simulink model "threeDOF"  (R2026a)
settings: Solver=FixedStepAuto  StopTime=30  FixedStep=0.01
settings Model: Creator=Lenovo  LastModifiedBy=Lenovo

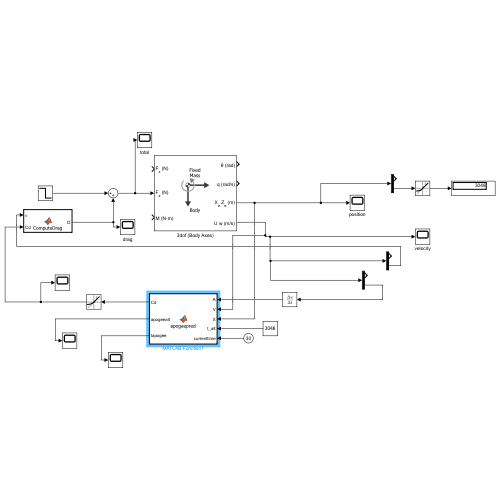
[thumbnail: Simulink's stored preview of the top-level diagram]
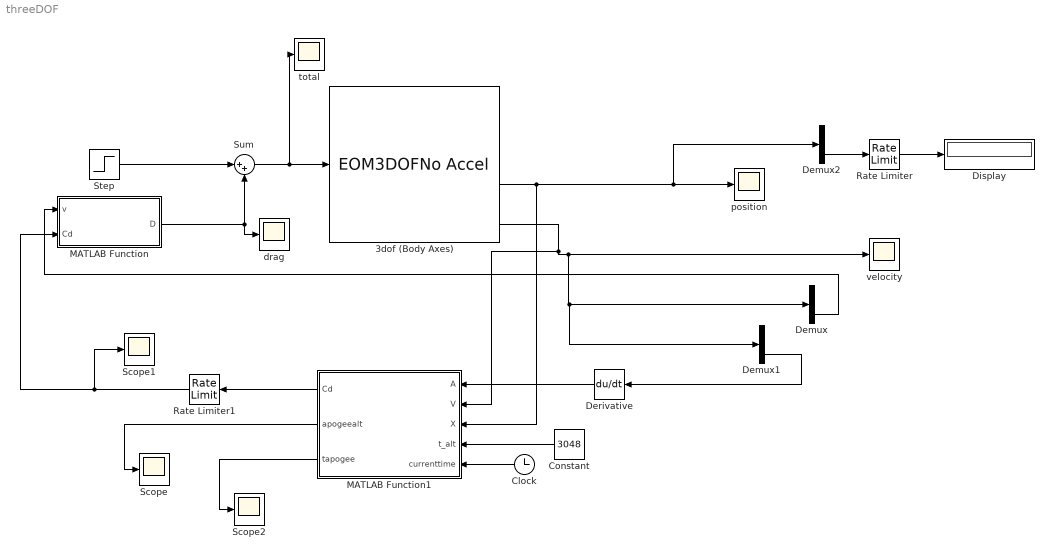
== system threeDOF ==
  3dof (Body Axes) : EOM3DOFNoAccel  v_ini=0  mass=19  g=-9.81
  Clock : Clock
  Constant : Constant  Value=3048
  Demux : Demux  Outputs=2
  Demux1 : Demux  Outputs=2
  Demux2 : Demux  Outputs=2
  Derivative : Derivative
  Display : Display
  MATLAB Function : MATLAB Function  TreatAsAtomicUnit=on
  MATLAB Function1 : MATLAB Function  TreatAsAtomicUnit=on
  Rate Limiter : RateLimiter  RisingSlewLimit=99999  FallingSlewLimit=0  SampleTimeMode=inherited
  Rate Limiter1 : RateLimiter  RisingSlewLimit=2  FallingSlewLimit=-2  SampleTimeMode=inherited
  Scope : Scope
      settings: ActiveDisplayYMinimum=-121.56338837946709  ActiveDisplayYMaximum=2234.7915316834028  DataLoggingVariableName=ScopeData4
  Scope1 : Scope
      settings: ActiveDisplayYMinimum=0.72031161367658469  ActiveDisplayYMaximum=0.76304547411750934  DataLoggingVariableName=ScopeData5
  Scope2 : Scope
      settings: ActiveDisplayYMinimum=-13.091307987348422  ActiveDisplayYMaximum=35.385913368142141  DataLoggingVariableName=ScopeData6
  Step : Step  Time=5.76  InitialValue=1152  FinalValue=0  SampleTime=0
  Sum : Sum  Inputs=|++
  drag : Scope
      settings: ActiveDisplayYMinimum=-396.86130675218692  ActiveDisplayYMaximum=62.412916979427223  DataLoggingVariableName=ScopeData2
  position : Scope
      settings: ActiveDisplayYMinimum=1923.5681768471607  ActiveDisplayYMaximum=4175.5644060181312
  total : Scope
      settings: ActiveDisplayYMinimum=-37.385165708014192  ActiveDisplayYMaximum=98.920743299033447  DataLoggingVariableName=ScopeData3
  velocity : Scope
      settings: ActiveDisplayYMinimum=-163.00745133948982  ActiveDisplayYMaximum=174.13780002379053
  wires:
  3dof (Body Axes)/3 -> MATLAB Function1/3(X), Demux2/1, position/1
  Step/1 -> Sum/1
  MATLAB Function/1(D) -> Sum/2, drag/1
  Sum/1 -> total/1, 3dof (Body Axes)/2
  3dof (Body Axes)/4 -> MATLAB Function1/2(V), Demux1/1, Demux/1, velocity/1
  Demux/2 -> MATLAB Function/1(v)
  Demux1/2 -> Derivative/1
  Derivative/1 -> MATLAB Function1/1(A)
  Constant/1 -> MATLAB Function1/4(t_alt)
  Clock/1 -> MATLAB Function1/5(currenttime)
  MATLAB Function1/1(Cd) -> Rate Limiter1/1
  Rate Limiter/1 -> Display/1
  Demux2/2 -> Rate Limiter/1
  Rate Limiter1/1 -> Scope1/1, MATLAB Function/2(Cd)
  MATLAB Function1/2(apogeealt) -> Scope/1
  MATLAB Function1/3(tapogee) -> Scope2/1

== matlab function threeDOF/MATLAB Function1 ==
  data: Cd output; apogeealt output; tapogee output; A input; V input; X input; t_alt input; currenttime input
function [Cd,apogeealt,tapogee] = apogeepred(A,V,X,t_alt,currenttime)

apogeeTG = t_alt;
currentAlt= X(2);
currentverticalvel=V(2);
currentverticalacc=A;

rho = 1.225;
Area = 0.018;
Cdclean = 0.3;
m = 19;
vsim = currentverticalvel;
altsim = currentAlt;
t = currenttime;
deltat = 0.01;
apogeealt = 0;
tapogee=0;

if(currentverticalacc > 0)
    Cd=Cdclean;
    return;
end

for c = 1:18
    Cdsim= Cdclean + c*0.03;
    for i = 1 : 3000
        F = -0.5*Cdsim*rho*Area*(vsim^2) - 9.81*m;

        asim= F/m;
        vsim = vsim + asim*deltat;
        altsim = altsim + vsim*deltat;
        t=t+deltat;

        if(vsim<0)
            apogeealt=altsim;
            tapogee = t;
            break;
        end

    end
    Cd=Cdsim;
    if apogeealt < apogeeTG
        break;
    end
end

== matlab function threeDOF/MATLAB Function ==
  data: v input; D output; Cd input
function D = ComputeDrag(v,Cd)
A=0.018;
rho = 1.225;
%Cd=0.3;

D = -0.25*Cd*rho*A*(v^2);
end
